simulink model "referenceTrackingModel"  (R2020b)
settings: Solver=VariableStepAuto  StartTime=0.0  StopTime=10.0  RelTol=1e-3
settings Model: Creator=kuzub  LastModifiedBy=kuzub

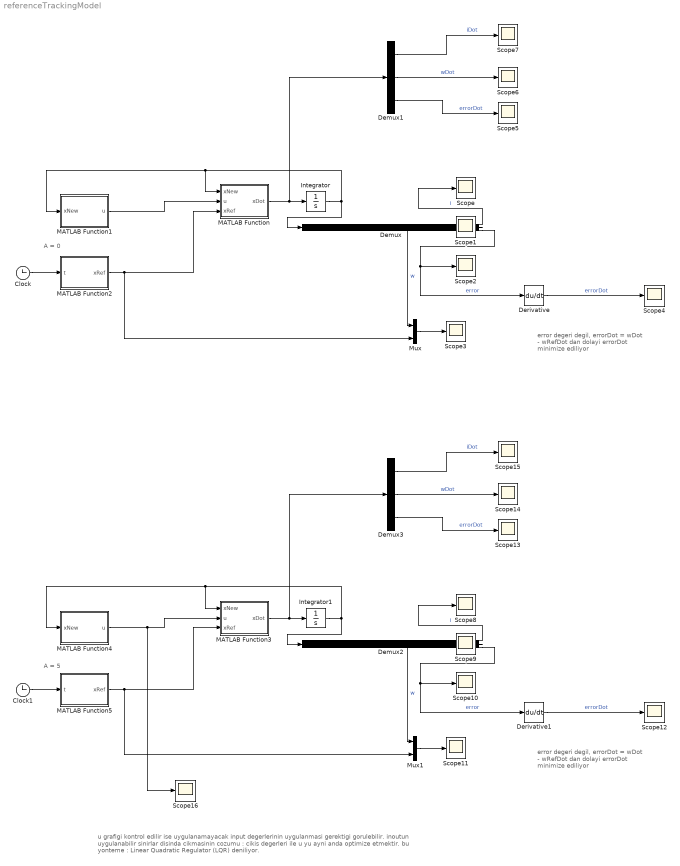
== system referenceTrackingModel ==
  note: u grafigi kontrol edilir ise uygulanamayacak input degerlerinin uygulanmasi gerektigi gorulebilir.
      |
      | inoutun uygulanabilir sinirlar disinda cikmasinin cozumu :
      | 	cikis degerleri ile u yu ayni anda optimize etmektir.
      |
      | bu yonteme : Linear Quadratic Regulator (LQR) deniliyor.
  note: A = 5
  note: error degeri degil,
      | errorDot = wDot - wRefDot
      | dan dolayi
      | errorDot minimize ediliyor
  note: error degeri degil,
      | errorDot = wDot - wRefDot
      | dan dolayi
      | errorDot minimize ediliyor
  note: A = 0
  Clock : Clock
  Clock1 : Clock
  Demux{,1..3} (4 alike) : Demux  Outputs=3
  Derivative : Derivative
  Derivative1 : Derivative
  Integrator : Integrator  InitialCondition=[0;0;0]
  Integrator1 : Integrator  InitialCondition=[0;0;0]
  MATLAB Function : MATLAB Function  TreatAsAtomicUnit=on
  MATLAB Function1 : MATLAB Function  TreatAsAtomicUnit=on
  MATLAB Function2 : MATLAB Function  TreatAsAtomicUnit=on
  MATLAB Function3 : MATLAB Function  TreatAsAtomicUnit=on
  MATLAB Function4 : MATLAB Function  TreatAsAtomicUnit=on
  MATLAB Function5 : MATLAB Function  TreatAsAtomicUnit=on
  Mux : Mux  Inputs=2
  Mux1 : Mux  Inputs=2
  Scope{,1..16} (17 alike) : Scope
  wires:
  MATLAB Function/1(xDot) -> Demux1/1, Integrator/1
  Integrator/1 -> MATLAB Function1/1(xNew), MATLAB Function/1(xNew), Demux/1
  MATLAB Function1/1(u) -> MATLAB Function/2(u)
  Clock/1 -> MATLAB Function2/1(t)
  MATLAB Function2/1(xRef) -> Mux/2, MATLAB Function/3(xRef)
  Demux/1 -> Scope/1  "i"
  Demux/3 -> Derivative/1, Scope2/1  "error"
  Demux/2 -> Mux/1, Scope1/1  "w"
  Mux/1 -> Scope3/1
  Derivative/1 -> Scope4/1  "errorDot"
  Demux1/3 -> Scope5/1  "errorDot"
  Demux1/1 -> Scope7/1  "iDot"
  Demux1/2 -> Scope6/1  "wDot"
  Demux3/2 -> Scope14/1  "wDot"
  Demux3/1 -> Scope15/1  "iDot"
  Demux3/3 -> Scope13/1  "errorDot"
  Derivative1/1 -> Scope12/1  "errorDot"
  Mux1/1 -> Scope11/1
  Demux2/2 -> Scope9/1, Mux1/1  "w"
  Demux2/3 -> Scope10/1, Derivative1/1  "error"
  Demux2/1 -> Scope8/1  "i"
  MATLAB Function5/1(xRef) -> MATLAB Function3/3(xRef), Mux1/2
  Clock1/1 -> MATLAB Function5/1(t)
  MATLAB Function4/1(u) -> Scope16/1, MATLAB Function3/2(u)
  Integrator1/1 -> Demux2/1, MATLAB Function3/1(xNew), MATLAB Function4/1(xNew)
  MATLAB Function3/1(xDot) -> Integrator1/1, Demux3/1

== matlab function referenceTrackingModel/MATLAB Function ==
  data: xNew input; u input; xDot output; xRef input
function xDot = fcn(xNew, u, xRef)
    %
    % Obtain all equation
    %
    % System Constants
    R = 0.55;
    J = 0.09;
    Kt = 85*10^-3;
    L = 25*10^-3;
    b = 0.05;
    %
    %% State Space Matrix
    %
    a00 = -R/L;
    a01 = -Kt/L;
    a10 = Kt/J;
    a11 = -b/J;
    %
    b00 = 1/L;
    b10 = 0;
    %
    A = [a00, a01;
         a10, a11];
    % 
    B = [b00; b10];
    %
    %% Reference Tracking 
    Anew = [A, zeros(2,1);
            0, 1, 0 ];
    %
    Bnew = [B; 0];
    %
    eRef = [0; 0; -1];


    xDot = Anew*xNew + Bnew*u + eRef*xRef;
end

== matlab function referenceTrackingModel/MATLAB Function2 ==
  data: t input; xRef output
function xRef = fcn(t)

    f = 0.1;
    A = 0;
    bias = 50;
    
    xRef = bias + A*sin(2*pi*f*t);

end

== matlab function referenceTrackingModel/MATLAB Function3 ==
  data: xNew input; u input; xDot output; xRef input
function xDot = fcn(xNew, u, xRef)
    %
    % Obtain all equation
    %
    % System Constants
    R = 0.55;
    J = 0.09;
    Kt = 85*10^-3;
    L = 25*10^-3;
    b = 0.05;
    %
    %% State Space Matrix
    %
    a00 = -R/L;
    a01 = -Kt/L;
    a10 = Kt/J;
    a11 = -b/J;
    %
    b00 = 1/L;
    b10 = 0;
    %
    A = [a00, a01;
         a10, a11];
    % 
    B = [b00; b10];
    %
    %% Reference Tracking 
    Anew = [A, zeros(2,1);
            0, 1, 0 ];
    %
    Bnew = [B; 0];
    %
    eRef = [0; 0; -1];


    xDot = Anew*xNew + Bnew*u + eRef*xRef;
end

== matlab function referenceTrackingModel/MATLAB Function4 ==
  data: xNew input; u output
function u = fcn(xNew)
    % Knew = [0.7361   21.9232  116.4706];
    Knew = (10^3)*[0.0043    0.3319    7.2265];
    u = -Knew*xNew;
end

== matlab function referenceTrackingModel/MATLAB Function5 ==
  data: t input; xRef output
function xRef = fcn(t)

    f = 0.1;
    A = 5;
    bias = 50;
    
    xRef = bias + A*sin(2*pi*f*t);

end

== matlab function referenceTrackingModel/MATLAB Function1 ==
  data: xNew input; u output
function u = fcn(xNew)
    % Knew = [0.7361   21.9232  116.4706];
    Knew = (10^3)*[0.0043    0.3319    7.2265];
    u = -Knew*xNew;
end
